simulink model "closedloop_simulink"  (R2020b)
settings: Solver=VariableStepAuto  StartTime=0.0  StopTime=0.007  RelTol=1e-3
values from neighbouring files (symbols this model uses):
  b = Trated / (Wrated * 2*pi / 60)    (= 0.0130454871387)    [closedloop_mat.m]    (also in openloop_mat.m)
  J = 0.0000071    (= 7.1e-06)    [closedloop_mat.m]    (also in openloop_mat.m)
  km = 0.0458    [closedloop_mat.m]    (also in openloop_mat.m)
  Lf = 2.63E-3    (= 0.00263)    [closedloop_mat.m]    (also in openloop_mat.m)
  n = 11.5    [closedloop_mat.m]    (also in openloop_mat.m)
  Rf = 2.49    [closedloop_mat.m]    (also in openloop_mat.m)
settings Model: Creator=Kevin Rim  LastModifiedBy=Kevin Rim

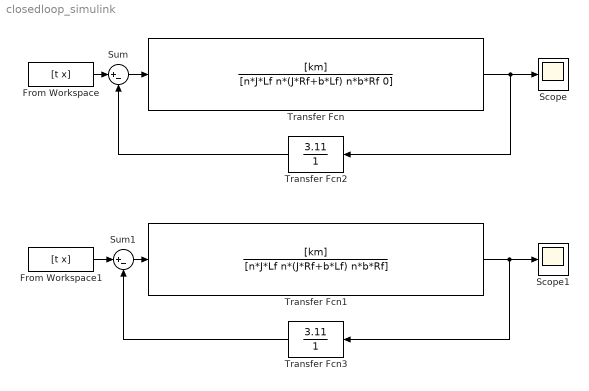
== system closedloop_simulink ==
  From Workspace : FromWorkspace  VariableName=[t x]  SampleTime=-1
  From Workspace1 : FromWorkspace  VariableName=[t x]  SampleTime=-1
  Scope : Scope
  Scope1 : Scope
  Sum : Sum  Inputs=|+-
  Sum1 : Sum  Inputs=|+-
  Transfer Fcn : TransferFcn  Numerator=[km]  Denominator=[n*J*Lf n*(J*Rf+b*Lf) n*b*Rf 0]
  Transfer Fcn1 : TransferFcn  Numerator=[km]  Denominator=[n*J*Lf n*(J*Rf+b*Lf) n*b*Rf]
  Transfer Fcn2 : TransferFcn  Numerator=[3.11]  Denominator=[1]
  Transfer Fcn3 : TransferFcn  Numerator=[3.11]  Denominator=[1]
  wires:
  From Workspace/1 -> Sum/1
  Transfer Fcn/1 -> Transfer Fcn2/1, Scope/1
  Sum/1 -> Transfer Fcn/1
  Transfer Fcn2/1 -> Sum/2
  Transfer Fcn3/1 -> Sum1/2
  From Workspace1/1 -> Sum1/1
  Sum1/1 -> Transfer Fcn1/1
  Transfer Fcn1/1 -> Transfer Fcn3/1, Scope1/1
